simulink model "stateSpaceController"  (R2015b)
settings: Solver=ode45  SolverMode=SingleTasking  StartTime=0.0  StopTime=4  RelTol=1e-3
values from neighbouring files (symbols this model uses):
  B_f = 7.7e-3    (= 0.0077)    [stateSpace.m]
  B_w = 17.03e-6    (= 1.703e-05)    [stateSpace.m]
  disturb = 0.65    [stateSpace.m]
  g = 9.82    [stateSpace.m]
  J_f = 4.8e-3    (= 0.0048)    [stateSpace.m]
  J_w = 0.601e-3    (= 0.000601)    [stateSpace.m]
  K = place(A,B,P)    [stateSpace.m]
  K1 = place(A,B,P1)    [stateSpace.m]
  l_f = 0.08498    [stateSpace.m]
  l_w = 0.093    [stateSpace.m]
  m_f = 0.77-m_w    (= 0.548)    [stateSpace.m]
  m_w = 0.222    [stateSpace.m]
  t_dist = 0.01    [stateSpace.m]
settings Model: Creator=USUARIO  LastModifiedBy=USUARIO
settings DataIOCC: SaveFormat=Array
settings OptimizationCC: BlockReduction=off  BooleanDataType=off
settings DebuggingCC: SaveWithParameterizedLinksMsg=none  UnderspecifiedInitializationDetection=Classic  MergeDetectMultiDrivingBlocksExec=none  SignalResolutionControl=TryResolveAllWithWarning
settings HardwareCC: ProdBitPerPointer=32  ProdLargestAtomicFloat=None  ProdIntDivRoundTo=Undefined  ProdEndianess=Unspecified  ProdWordSize=32  ProdHWDeviceType=32-bit Generic  TargetUnknown=on
settings GRTTargetCC: GeneratePreprocessorConditionals=Disable all
settings ConfigComp: CovModelRefEnable=Off  CovSFcnEnable=off

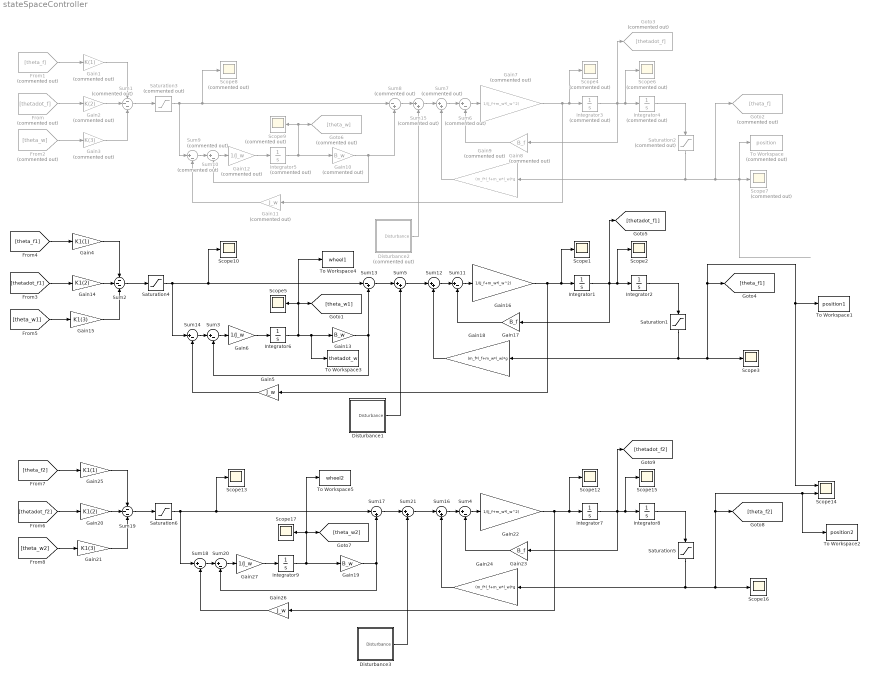
== system stateSpaceController ==
  Disturbance1 : Subsystem
  Disturbance2 : Subsystem  Commented=on
  Disturbance3 : Subsystem
  From : From  Commented=on  GotoTag=thetadot_f
  From1 : From  Commented=on  GotoTag=theta_f
  From2 : From  Commented=on  GotoTag=theta_w
  Gain1 : Gain  Commented=on  Gain=K(1)
  Gain10 : Gain  Commented=on  Gain=B_w
  Gain11 : Gain  Commented=on  Gain=J_w
  Gain12 : Gain  Commented=on  Gain=1/J_w
  Gain13 : Gain  Gain=B_w
  Gain14 : Gain  Gain=K1(2)
  Gain15 : Gain  Gain=K1(3)
  Gain16 : Gain  Gain=1/(J_f+m_w*l_w^2)
  Gain17 : Gain  Gain=B_f
  Gain18 : Gain  Gain=(m_f*l_f+m_w*l_w)*g
  Gain19 : Gain  Gain=B_w
  Gain2 : Gain  Commented=on  Gain=K(2)
  Gain20 : Gain  Gain=K1(2)
  Gain21 : Gain  Gain=K1(3)
  Gain22 : Gain  Gain=1/(J_f+m_w*l_w^2)
  Gain23 : Gain  Gain=B_f
  Gain24 : Gain  Gain=(m_f*l_f+m_w*l_w)*g
  Gain25 : Gain  Gain=K1(1)
  Gain26 : Gain  Gain=J_w
  Gain27 : Gain  Gain=1/J_w
  Gain3 : Gain  Commented=on  Gain=K(3)
  Gain4 : Gain  Gain=K1(1)
  Gain5 : Gain  Gain=J_w
  Gain6 : Gain  Gain=1/J_w
  Gain7 : Gain  Commented=on  Gain=1/(J_f+m_w*l_w^2)
  Gain8 : Gain  Commented=on  Gain=B_f
  Gain9 : Gain  Commented=on  Gain=(m_f*l_f+m_w*l_w)*g
  Goto2 : Goto  Commented=on  GotoTag=theta_f
  Goto3 : Goto  Commented=on  GotoTag=thetadot_f
  Goto6 : Goto  Commented=on  GotoTag=theta_w
  Integrator1 : Integrator  InitialCondition=1.57
  Integrator2 : Integrator  InitialCondition=-0.2
  Integrator3 : Integrator  Commented=on  InitialCondition=1.57
  Integrator4 : Integrator  Commented=on  InitialCondition=-0.2
  Integrator5 : Integrator  Commented=on
  Integrator{6..9} (4 alike) : Integrator
  Saturation1 : Saturate  UpperLimit=0.85  LowerLimit=-0.72
  Saturation2 : Saturate  Commented=on  UpperLimit=0.85  LowerLimit=-0.72
  Saturation3 : Saturate  Commented=on  UpperLimit=4*0.0335  LowerLimit=-4*0.0335
  Saturation4 : Saturate  UpperLimit=4*0.0335  LowerLimit=-4*0.0335
  Saturation5 : Saturate  UpperLimit=0.85  LowerLimit=-0.72
  Saturation6 : Saturate  UpperLimit=4*0.0335  LowerLimit=-4*0.0335
  Scope{1..3,5,10,12..13,15..17} (10 alike) : Scope
  Scope14 : Scope  NumInputPorts=2
  Scope{4,6..9} (5 alike) : Scope  Commented=on
  Sum1 : Sum  Commented=on  Inputs=---
  Sum10 : Sum  Commented=on  Inputs=|+-
  Sum{3..4,11,14,18,20} (6 alike) : Sum  Inputs=|+-
  Sum{5,12,16,21} (4 alike) : Sum  Inputs=|++
  Sum13 : Sum  Inputs=|-+
  Sum15 : Sum  Commented=on  Inputs=|++
  Sum17 : Sum  Inputs=|-+
  Sum19 : Sum  Inputs=---
  Sum2 : Sum  Inputs=---
  Sum6 : Sum  Commented=on  Inputs=|+-
  Sum7 : Sum  Commented=on  Inputs=|++
  Sum8 : Sum  Commented=on  Inputs=|-+
  Sum9 : Sum  Commented=on  Inputs=|+-
  To Workspace : ToWorkspace  Commented=on  VariableName=position  SaveFormat=Timeseries  SampleTime=-1
  To Workspace1 : ToWorkspace  VariableName=position1  SaveFormat=Timeseries  SampleTime=-1
  To Workspace2 : ToWorkspace  VariableName=position2  SaveFormat=Timeseries  SampleTime=-1
  To Workspace3 : ToWorkspace  VariableName=thetadot_w  SaveFormat=Timeseries  SampleTime=-1
  To Workspace4 : ToWorkspace  VariableName=wheel1  SaveFormat=Timeseries  SampleTime=-1
  To Workspace5 : ToWorkspace  VariableName=wheel2  SaveFormat=Timeseries  SampleTime=-1
  wires:
  Gain7/1 -> Gain11/1, Scope4/1, Integrator3/1
  Integrator3/1 -> Goto3/1, Gain8/1, Scope6/1, Integrator4/1
  Sum6/1 -> Gain7/1
  Sum7/1 -> Sum6/1
  Gain8/1 -> Sum6/2
  Gain9/1 -> Sum7/2
  Integrator4/1 -> Saturation2/1
  Sum1/1 -> Saturation3/1
  From1/1 -> Gain1/1
  From/1 -> Gain2/1
  From2/1 -> Gain3/1
  Gain1/1 -> Sum1/1
  Gain3/1 -> Sum1/3
  Gain2/1 -> Sum1/2
  Saturation2/1 -> Gain9/1, Goto2/1, Scope7/1, To Workspace/1
  Gain16/1 -> Gain5/1, Scope1/1, Integrator1/1
  Integrator1/1 -> [thetadot_f1], Gain17/1, Scope2/1, Integrator2/1
  Sum11/1 -> Gain16/1
  Sum12/1 -> Sum11/1
  Gain17/1 -> Sum11/2
  Gain18/1 -> Sum12/2
  Sum3/1 -> Gain6/1
  Gain6/1 -> Integrator6/1
  Gain5/1 -> Sum14/2
  Sum14/1 -> Sum3/1
  Integrator6/1 -> To Workspace3/1, Gain13/1, To Workspace4/1, Scope5/1, [theta_w1]
  Gain13/1 -> Sum3/2, Sum13/2
  Integrator2/1 -> Saturation1/1
  Saturation4/1 -> Sum14/1, Sum13/1, Scope10/1
  Sum2/1 -> Saturation4/1
  [theta_f1] -> Gain4/1
  [thetadot_f1] -> Gain14/1
  [theta_w1] -> Gain15/1
  Gain4/1 -> Sum2/1
  Gain15/1 -> Sum2/3
  Gain14/1 -> Sum2/2
  Saturation1/1 -> Gain18/1, Scope14/1, To Workspace1/1, [theta_f1], Scope3/1
  Disturbance1/1(Disturbance) -> Sum5/2
  Sum13/1 -> Sum5/1
  Sum5/1 -> Sum12/1
  Sum10/1 -> Gain12/1
  Gain12/1 -> Integrator5/1
  Gain11/1 -> Sum9/2
  Sum9/1 -> Sum10/1
  Integrator5/1 -> Gain10/1, Scope9/1, Goto6/1
  Gain10/1 -> Sum10/2, Sum8/2
  Saturation3/1 -> Sum9/1, Sum8/1, Scope8/1
  Disturbance2/1(Disturbance) -> Sum15/2
  Sum8/1 -> Sum15/1
  Sum15/1 -> Sum7/1
  Gain22/1 -> Gain26/1, Scope12/1, Integrator7/1
  Integrator7/1 -> [thetadot_f2], Gain23/1, Scope15/1, Integrator8/1
  Sum4/1 -> Gain22/1
  Sum16/1 -> Sum4/1
  Gain23/1 -> Sum4/2
  Gain24/1 -> Sum16/2
  Sum20/1 -> Gain27/1
  Gain27/1 -> Integrator9/1
  Gain26/1 -> Sum18/2
  Sum18/1 -> Sum20/1
  Integrator9/1 -> Gain19/1, To Workspace5/1, Scope17/1, [theta_w2]
  Gain19/1 -> Sum20/2, Sum17/2
  Integrator8/1 -> Saturation5/1
  Saturation6/1 -> Sum18/1, Sum17/1, Scope13/1
  Sum19/1 -> Saturation6/1
  [theta_f2] -> Gain25/1
  [thetadot_f2] -> Gain20/1
  [theta_w2] -> Gain21/1
  Gain25/1 -> Sum19/1
  Gain21/1 -> Sum19/3
  Gain20/1 -> Sum19/2
  Saturation5/1 -> Gain24/1, To Workspace2/1, Scope14/2, [theta_f2], Scope16/1
  Disturbance3/1(Disturbance) -> Sum21/2
  Sum17/1 -> Sum21/1
  Sum21/1 -> Sum16/1

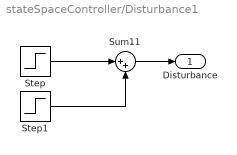
== system stateSpaceController/Disturbance1 ==
  Step : Step  Time=0.1  After=disturb  SampleTime=0
  Step1 : Step  Time=0.1+t_dist  After=-disturb  SampleTime=0
  Sum11 : Sum  Inputs=|++
  Disturbance : Outport
  wires:
  Step1/1 -> Sum11/2
  Step/1 -> Sum11/1
  Sum11/1 -> Disturbance/1

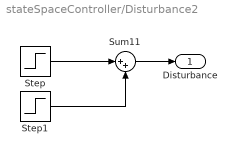
== system stateSpaceController/Disturbance2 ==
  Step : Step  Time=0.1  After=disturb  SampleTime=0
  Step1 : Step  Time=0.1+t_dist  After=-disturb  SampleTime=0
  Sum11 : Sum  Inputs=|++
  Disturbance : Outport
  wires:
  Step1/1 -> Sum11/2
  Step/1 -> Sum11/1
  Sum11/1 -> Disturbance/1

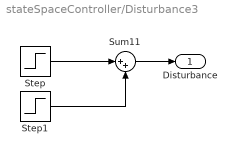
== system stateSpaceController/Disturbance3 ==
  Step : Step  Time=0.1  After=disturb  SampleTime=0
  Step1 : Step  Time=0.1+t_dist  After=-disturb  SampleTime=0
  Sum11 : Sum  Inputs=|++
  Disturbance : Outport
  wires:
  Step1/1 -> Sum11/2
  Step/1 -> Sum11/1
  Sum11/1 -> Disturbance/1
